simulink model "Controller"  (R2017b)
settings: Solver=VariableStepAuto  StartTime=0.0  StopTime=10.0  RelTol=1e-3
values from neighbouring files (symbols this model uses):
  A = [0          1                        0                0 ... (first row only)    [InvertedPendulum.m]
  B = [0; 4/(4*M+m); 0; 3/(4*M*l+m*l)]    [InvertedPendulum.m]
  C = [1 0 0 0; 0 0 1 0]    [InvertedPendulum.m]
  K = acker(A, B, P)    [InvertedPendulum.m]
settings Model: Creator=Daniel Ramos  LastModifiedBy=Daniel Ramos

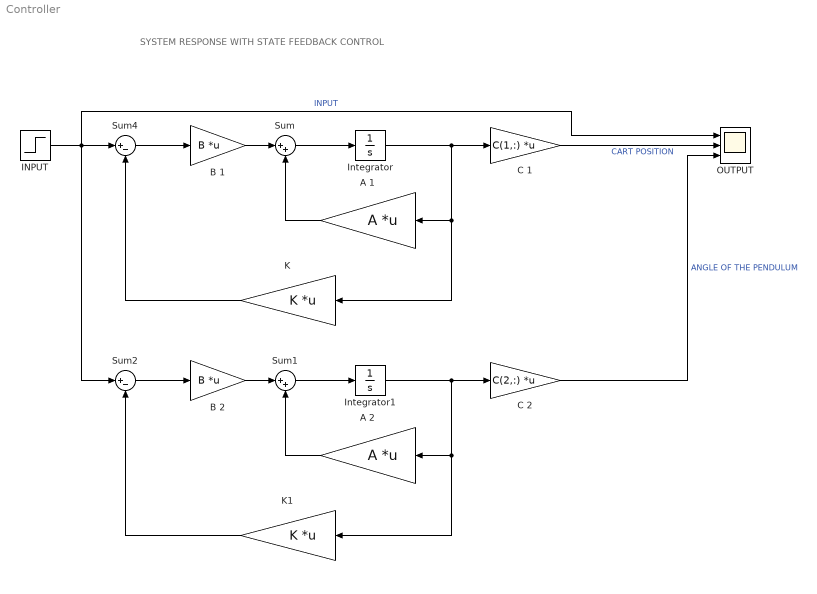
== system Controller ==
  note: SYSTEM RESPONSE WITH STATE FEEDBACK CONTROL
  A 1 : Gain  Gain=A  Multiplication=Matrix(K*u)
  A 2 : Gain  Gain=A  Multiplication=Matrix(K*u)
  B 1 : Gain  Gain=B  Multiplication=Matrix(K*u)
  B 2 : Gain  Gain=B  Multiplication=Matrix(K*u)
  C 1 : Gain  Gain=C(1,:)  Multiplication=Matrix(K*u)
  C 2 : Gain  Gain=C(2,:)  Multiplication=Matrix(K*u)
  INPUT : Step  Time=0  SampleTime=0
  Integrator : Integrator
  Integrator1 : Integrator
  K : Gain  Gain=K  Multiplication=Matrix(K*u)
  K1 : Gain  Gain=K  Multiplication=Matrix(K*u)
  OUTPUT : Scope  NumInputPorts=3
  Sum : Sum  Inputs=|++
  Sum1 : Sum  Inputs=|++
  Sum2 : Sum  Inputs=|+-
  Sum4 : Sum  Inputs=|+-
  wires:
  Sum/1 -> Integrator/1
  Integrator/1 -> K/1, A 1/1, C 1/1
  B 1/1 -> Sum/1
  A 1/1 -> Sum/2
  C 1/1 -> OUTPUT/2  "CART POSITION"
  Sum4/1 -> B 1/1
  K/1 -> Sum4/2
  INPUT/1 -> Sum2/1, OUTPUT/1, Sum4/1  "INPUT"
  K1/1 -> Sum2/2
  Integrator1/1 -> K1/1, A 2/1, C 2/1
  B 2/1 -> Sum1/1
  Sum2/1 -> B 2/1
  A 2/1 -> Sum1/2
  Sum1/1 -> Integrator1/1
  C 2/1 -> OUTPUT/3  "ANGLE OF THE PENDULUM"
